simulink model "pres2"  (R2020a)
settings: Solver=FixedStepAuto  StartTime=0.0  StopTime=10.0  FixedStep=0.001  RelTol=1e-3
undefined symbols (not defined in the file): c1, c2, c3, Ca, Cv, Ed, Es0, omega0, Ra, Rlv, Rv, T, Tsys
libraries: simulink x1
settings Model: Creator=sebastian  LastModifiedBy=luisi

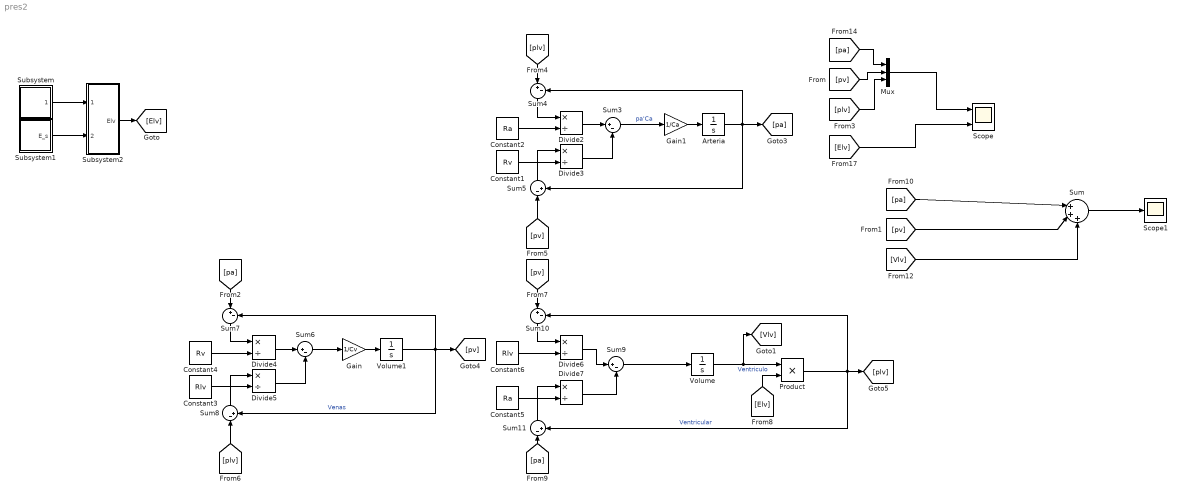
== system pres2 ==
  Arteria : Integrator
  Constant1 : Constant  Value=Rv
  Constant2 : Constant  Value=Ra
  Constant3 : Constant  Value=Rlv
  Constant4 : Constant  Value=Rv
  Constant5 : Constant  Value=Ra
  Constant6 : Constant  Value=Rlv
  Divide{2..7} (6 alike) : Product  Inputs=*/
  Gain : Gain  Gain=1/Cv
  Gain1 : Gain  Gain=1/Ca
  Mux : Mux  Inputs=3
  Product : Product
  Scope : Scope  NumInputPorts=2
  Scope1 : Scope
  Subsystem : Subsystem
  Subsystem1 : Subsystem
  Subsystem2 : Subsystem
  Sum : Sum  Inputs=|+++
  Sum{3..4,6..7,9..10} (6 alike) : Sum  Inputs=|+-
  Sum11 : Sum  Inputs=|-+
  Sum5 : Sum  Inputs=|-+
  Sum8 : Sum  Inputs=|-+
  Volume : Integrator  InitialCondition=17
  Volume1 : Integrator  InitialCondition=90
  wires:
  Divide6/1 -> Sum9/1
  Divide5/1 -> Sum6/2
  Constant6/1 -> Divide6/2
  Sum6/1 -> Gain/1
  Sum5/1 -> Divide3/1
  Sum8/1 -> Divide5/1
  Product/1 -> Sum10/2, [plv], Sum11/2  "Ventricular"
  [plv] -> Sum8/1
  [pv] -> Sum10/1
  Constant2/1 -> Divide2/2
  Sum11/1 -> Divide7/1
  Constant5/1 -> Divide7/2
  Sum4/1 -> Divide2/1
  Subsystem2/1(Elv) -> [Elv]
  [Elv] -> Scope/2
  Divide2/1 -> Sum3/1
  Constant1/1 -> Divide3/2
  Divide7/1 -> Sum9/2
  [plv] -> Sum4/1
  Arteria/1 -> Sum5/2, Sum4/2, [pa]
  Sum3/1 -> Gain1/1  "pa'Ca"
  Constant3/1 -> Divide5/2
  Subsystem1/1(E_s) -> Subsystem2/2(E_s)
  Divide4/1 -> Sum6/1
  Constant4/1 -> Divide4/2
  [pv] -> Sum5/1
  Sum10/1 -> Divide6/1
  Divide3/1 -> Sum3/2
  Sum7/1 -> Divide4/1
  [pa] -> Sum11/1
  Subsystem/1(alpha_t) -> Subsystem2/1(alpha)
  [pa] -> Sum7/1
  Sum9/1 -> Volume/1
  [Elv] -> Product/2
  Volume/1 -> [Vlv], Product/1  "Ventriculo"
  [pa] -> Mux/1
  [pv] -> Mux/2
  [plv] -> Mux/3
  Mux/1 -> Scope/1
  Sum/1 -> Scope1/1
  Volume1/1 -> [pv], Sum8/2, Sum7/2  "Venas"
  Gain/1 -> Volume1/1
  Gain1/1 -> Arteria/1
  [Vlv] -> Sum/3
  [pa] -> Sum/1
  [pv] -> Sum/2

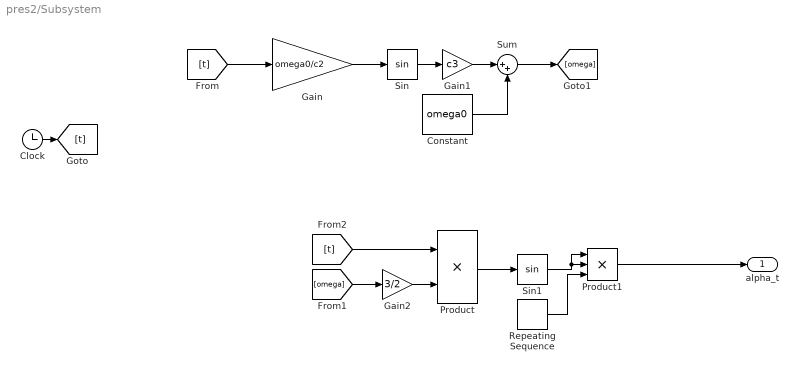
== system pres2/Subsystem ==
  Clock : Clock
  Constant : Constant  Value=omega0
  Gain : Gain  Gain=omega0/c2
  Gain1 : Gain  Gain=c3
  Gain2 : Gain  Gain=3/2
  Product : Product
  Product1 : Product  Inputs=3
  Repeating Sequence : simulink/Sources/Repeating Sequence  rep_seq_t=[0 Tsys Tsys+0.001 T]  rep_seq_y=[1 1 0 0]
  Sin : Trigonometry
  Sin1 : Trigonometry
  Sum : Sum  Inputs=|++
  alpha_t : Outport
  wires:
  Clock/1 -> [t]
  [t] -> Gain/1
  Gain/1 -> Sin/1
  Sin/1 -> Gain1/1
  Gain1/1 -> Sum/1
  Constant/1 -> Sum/2
  Sum/1 -> [omega]
  [t] -> Product/1
  [omega] -> Gain2/1
  Product/1 -> Sin1/1
  Sin1/1 -> Product1/1, Product1/2
  Product1/1 -> alpha_t/1
  Gain2/1 -> Product/2
  Repeating Sequence/1 -> Product1/3

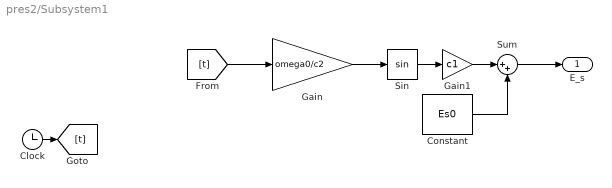
== system pres2/Subsystem1 ==
  Clock : Clock
  Constant : Constant  Value=Es0
  Gain : Gain  Gain=omega0/c2
  Gain1 : Gain  Gain=c1
  Sin : Trigonometry
  Sum : Sum  Inputs=|++
  E_s : Outport
  wires:
  Sum/1 -> E_s/1
  Constant/1 -> Sum/2
  Gain1/1 -> Sum/1
  Sin/1 -> Gain1/1
  Gain/1 -> Sin/1
  [t] -> Gain/1
  Clock/1 -> [t]

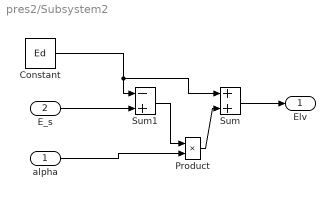
== system pres2/Subsystem2 ==
  alpha : Inport
  E_s : Inport  Port=2
  Constant : Constant  Value=Ed
  Product : Product
  Sum : Sum
  Sum1 : Sum  Inputs=-+
  Elv : Outport
  wires:
  Constant/1 -> Sum1/1, Sum/1
  E_s/1 -> Sum1/2
  alpha/1 -> Product/2
  Sum1/1 -> Product/1
  Product/1 -> Sum/2
  Sum/1 -> Elv/1
